simulink model "simulation"  (R2023b)
settings: Solver=FixedStepAuto  StartTime=0.0  StopTime=1e-6  FixedStep=1e-9  RelTol=1e-3
undefined symbols (not defined in the file): sigbuilder_block
libraries: fl_lib x47, nesl_utility x9, ee_lib x8
settings Model: Creator=Ryan  LastModifiedBy=shenjiarun
settings SolverCC: AlgebraicLoopSolver=TrustRegion
settings DebuggingCC: UnconnectedInputMsg=warning  UnconnectedOutputMsg=warning  UnconnectedLineMsg=warning
settings ModelReferenceCC: EnableRefExpFcnMdlSchedulingChecks=on
settings SFSimCC: CustomCodeUndefinedFunction=UseInterfaceOnly

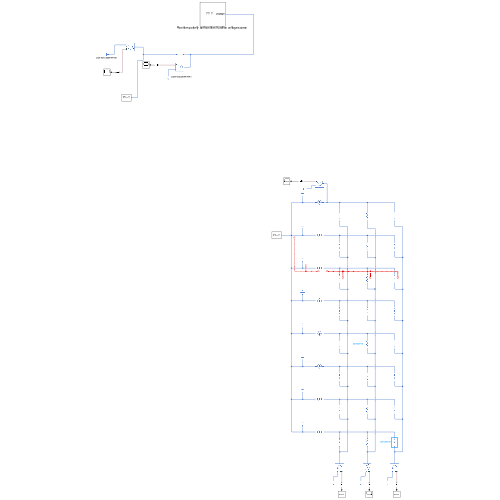
[thumbnail: Simulink's stored preview of the top-level diagram]
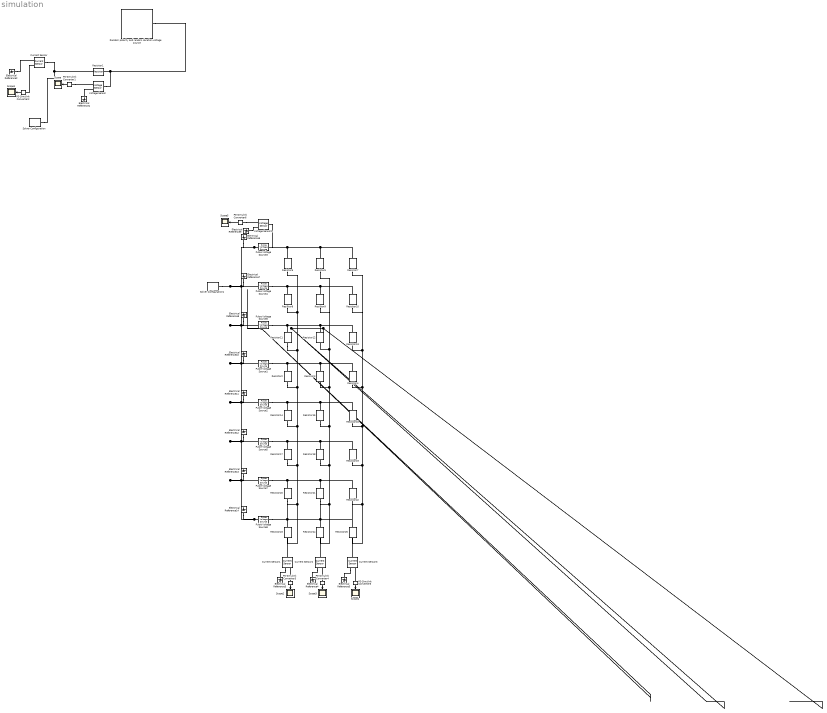
== system simulation ==
  Current Sensor{,1..3} (4 alike) : fl_lib/Electrical/Electrical Sensors/Current Sensor
  Electrical Reference{1..14} (14 alike) : fl_lib/Electrical/Electrical Elements/Electrical Reference
  PS-Simulink Converter{1..6} (6 alike) : nesl_utility/PS-Simulink Converter  PhysicalDomain=network_engine_domain  SubClassName=ps_output  LeftPortType=input  RightPortType=output  PseudoPeriodic=off  Frequencies=[]  VectorFormat=1-D array  Unit=1  AffineConversion=off
  Pulse Voltage Source{1,3,6,8} (4 alike) : ee_lib/Additional Components/SPICE Sources/Pulse Voltage Source  V1=0 V  V2=0.008 V  TD=0 s  TR=1e-9 s  TF=1e-9 s  PW=500e-9 s  PER=inf s
      settings: InternalSimscapePortConfiguration="{\"Bottom\":[],\"Left\":[{\"id\":\"p\",\"label\":\"\",\"type\":\"foundation.electrical.electrical\"}],\"Right\":[{\"id\":\"n\",\"label\":\"\",\"type\":\"foundation.electrical.electrical\"}],\"Top\":[]}"
  Pulse Voltage Source{2,4..5,7} (4 alike) : ee_lib/Additional Components/SPICE Sources/Pulse Voltage Source  V1=0 V  V2=0.2 V  TD=0 s  TR=1e-9 s  TF=1e-9 s  PW=500e-9 s  PER=inf s
      settings: InternalSimscapePortConfiguration="{\"Bottom\":[],\"Left\":[{\"id\":\"p\",\"label\":\"\",\"type\":\"foundation.electrical.electrical\"}],\"Right\":[{\"id\":\"n\",\"label\":\"\",\"type\":\"foundation.electrical.electrical\"}],\"Top\":[]}"
  Random polarity and random duration voltage source : Subsystem
      mask Display: image('D:\BaiduSyncdisk\UESTC\2022忆阻器萤火虫算法\论文写作\crossbar\随机.png');
  Resistor{1..3,5,7,9..11,13,16,18..19,22..25} (16 alike) : fl_lib/Electrical/Electrical Elements/Resistor  R=100 Ohm  i_specify=off  i_priority=None  i=0 A  i_nominal_specify=off  i_nominal_unit=A  i_nominal_value=1  v_specify=off  v_priority=None  v=0 V  v_nominal_specify=off  v_nominal_unit=V  v_nominal_value=1
  Resistor{4,6,8,12,14..15,17,20..21} (9 alike) : fl_lib/Electrical/Electrical Elements/Resistor  R=2500 Ohm  i_specify=off  i_priority=None  i=0 A  i_nominal_specify=off  i_nominal_unit=A  i_nominal_value=1  v_specify=off  v_priority=None  v=0 V  v_nominal_specify=off  v_nominal_unit=V  v_nominal_value=1
  Scope{,1..5} (6 alike) : Scope
  Solver Configuration : nesl_utility/Solver Configuration  PhysicalDomain=network_engine_domain  SubClassName=solver  LeftPortType=input  RightPortType=generic  Tones=[]  Harmonics=[]  SimulateNoise=off  Profile=off  UseLocalSampling=off  EnableSwitchedLinearOptims=on  FrequencyDomain=off  UseCCode=off  RelTol=0.001  AbsTol=1e-06  MinStep=1e-09  ToWorkspace=off  RevertToSquareIcSolve=off  NumHomotopyIterations=100  PhasorMode=off  PhasorModeNumHarmonics=1  ConsistencySolver=NEWTON_FTOL  IndexReductionMethod=DerivativeReplacement  DoDC=off  ResidualTolerance=1e-09  ConsistencyTolSource=GLOBAL  ConsistencyAbsTol=0.001  ConsistencyRelTol=0.001  ConsistencyTolFactor=0.001  UseLocalSolver=off  LocalSolverChoice=NE_BACKWARD_EULER_ADVANCER  ResolveIndetEquations=on  FunctionEvalNumThread=1  LocalSolverSampleTime=0.001  DoFixedCost=off  MaxNonlinIter=3  MaxModeIter=2  ComputeImpulses=off  ImpulseIterations=2  LinearAlgebra=auto  LinearAlgebraNumThread=0  EquationFormulation=NE_TIME_EF  DelaysMemoryBudget=1024  AutomaticFiltering=on  FilteringTimeConstant=0.001  PartitionStorageMethod=AS_NEEDED  PartitionMemoryBudget=1024  PartitionMethod=ROBUST  MultibodyUseLocalSolver=off  MultibodyLocalSolverChoice=ODE1  MultibodyLocalSolverSampleTime=0.001
  Solver Configuration1 : nesl_utility/Solver Configuration  PhysicalDomain=network_engine_domain  SubClassName=solver  LeftPortType=input  RightPortType=generic  Tones=[]  Harmonics=[]  SimulateNoise=off  Profile=off  UseLocalSampling=off  EnableSwitchedLinearOptims=on  FrequencyDomain=off  UseCCode=off  RelTol=0.001  AbsTol=1e-06  MinStep=1e-09  ToWorkspace=off  RevertToSquareIcSolve=off  NumHomotopyIterations=100  PhasorMode=off  PhasorModeNumHarmonics=1  ConsistencySolver=NEWTON_FTOL  IndexReductionMethod=DerivativeReplacement  DoDC=off  ResidualTolerance=1e-09  ConsistencyTolSource=GLOBAL  ConsistencyAbsTol=0.001  ConsistencyRelTol=0.001  ConsistencyTolFactor=0.001  UseLocalSolver=off  LocalSolverChoice=NE_BACKWARD_EULER_ADVANCER  ResolveIndetEquations=on  FunctionEvalNumThread=1  LocalSolverSampleTime=0.001  DoFixedCost=off  MaxNonlinIter=3  MaxModeIter=2  ComputeImpulses=off  ImpulseIterations=2  LinearAlgebra=auto  LinearAlgebraNumThread=0  EquationFormulation=NE_TIME_EF  DelaysMemoryBudget=1024  AutomaticFiltering=on  FilteringTimeConstant=0.001  PartitionStorageMethod=AS_NEEDED  PartitionMemoryBudget=1024  PartitionMethod=ROBUST  MultibodyUseLocalSolver=off  MultibodyLocalSolverChoice=ODE1  MultibodyLocalSolverSampleTime=0.001
  Voltage Sensor : fl_lib/Electrical/Electrical Sensors/Voltage Sensor
  Voltage Sensor1 : fl_lib/Electrical/Electrical Sensors/Voltage Sensor
  wires:
  PS-Simulink Converter1/1 -> Scope/1
  PS-Simulink Converter2/1 -> Scope1/1
  PS-Simulink Converter5/1 -> Scope4/1
  PS-Simulink Converter3/1 -> Scope2/1
  PS-Simulink Converter4/1 -> Scope3/1
  PS-Simulink Converter6/1 -> Scope5/1
  connections:
  Random polarity and random duration voltage source/RConn1 -- Voltage Sensor/LConn1 -- Resistor1/LConn1
  Solver Configuration/RConn1 -- Current Sensor/LConn1 -- Resistor1/RConn1
  Electrical Reference1/LConn1 -- Voltage Sensor/RConn2
  PS-Simulink Converter1/LConn1 -- Voltage Sensor/RConn1
  Electrical Reference2/LConn1 -- Current Sensor/RConn2
  PS-Simulink Converter2/LConn1 -- Current Sensor/RConn1
  Pulse Voltage Source8/RConn1 -- Solver Configuration1/RConn1 -- Electrical Reference7/LConn1 -- Pulse Voltage Source4/RConn1 -- Pulse Voltage Source3/RConn1 -- Electrical Reference6/LConn1 -- Electrical Reference8/LConn1 -- Pulse Voltage Source6/RConn1 -- Electrical Reference10/LConn1 -- Pulse Voltage Source1/RConn1 -- Electrical Reference11/LConn1 -- Pulse Voltage Source2/RConn1 -- Electrical Reference12/LConn1 -- Pulse Voltage Source5/RConn1 -- Electrical Reference13/LConn1 -- Pulse Voltage Source7/RConn1 -- Electrical Reference14/LConn1
  Resistor13/LConn1 -- Pulse Voltage Source6/LConn1 -- Resistor11/LConn1 -- Resistor12/LConn1
  Resistor6/LConn1 -- Resistor7/LConn1 -- Voltage Sensor1/LConn1 -- Pulse Voltage Source3/LConn1 -- Resistor5/LConn1
  Resistor9/LConn1 -- Resistor10/LConn1 -- Pulse Voltage Source4/LConn1 -- Resistor8/LConn1
  Resistor10/RConn1 -- Resistor7/RConn1 -- Current Sensor3/LConn1 -- Resistor25/RConn1 -- Resistor22/RConn1 -- Resistor19/RConn1 -- Resistor16/RConn1 -- Resistor4/RConn1 -- Resistor13/RConn1
  Resistor5/RConn1 -- Current Sensor1/LConn1 -- Resistor23/RConn1 -- Resistor20/RConn1 -- Resistor17/RConn1 -- Resistor14/RConn1 -- Resistor2/RConn1 -- Resistor11/RConn1 -- Resistor8/RConn1
  Resistor9/RConn1 -- Resistor6/RConn1 -- Current Sensor2/LConn1 -- Resistor24/RConn1 -- Resistor21/RConn1 -- Resistor18/RConn1 -- Resistor15/RConn1 -- Resistor3/RConn1 -- Resistor12/RConn1
  PS-Simulink Converter5/LConn1 -- Current Sensor3/RConn1
  PS-Simulink Converter3/LConn1 -- Current Sensor1/RConn1
  Current Sensor3/RConn2 -- Electrical Reference5/LConn1
  Current Sensor2/RConn2 -- Electrical Reference4/LConn1
  Current Sensor1/RConn2 -- Electrical Reference3/LConn1
  PS-Simulink Converter4/LConn1 -- Current Sensor2/RConn1
  Electrical Reference9/LConn1 -- Voltage Sensor1/RConn2
  PS-Simulink Converter6/LConn1 -- Voltage Sensor1/RConn1
  Resistor3/LConn1 -- Resistor4/LConn1 -- Pulse Voltage Source1/LConn1 -- Resistor2/LConn1
  Resistor15/LConn1 -- Resistor16/LConn1 -- Pulse Voltage Source2/LConn1 -- Resistor14/LConn1
  Resistor18/LConn1 -- Resistor19/LConn1 -- Pulse Voltage Source5/LConn1 -- Resistor17/LConn1
  Resistor21/LConn1 -- Resistor22/LConn1 -- Pulse Voltage Source7/LConn1 -- Resistor20/LConn1
  Resistor24/LConn1 -- Resistor25/LConn1 -- Pulse Voltage Source8/LConn1 -- Resistor23/LConn1
  ?
  ?
  ?
  ?
  ?
  ?

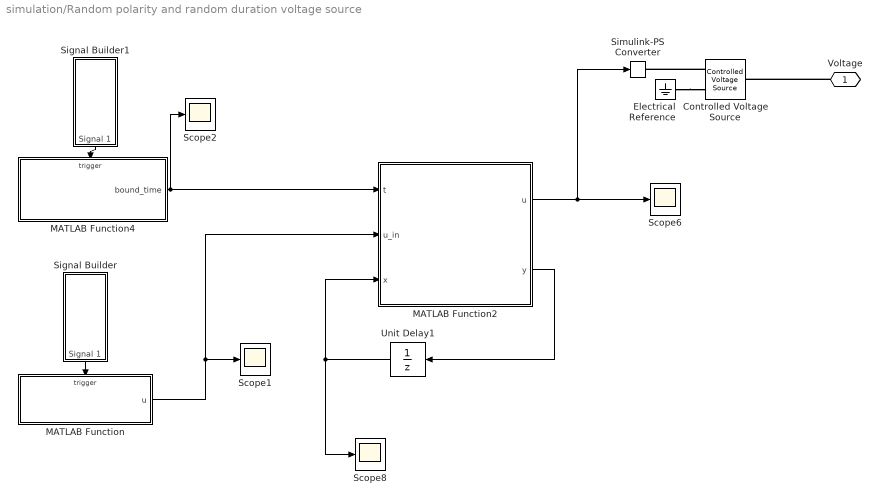
== system simulation/Random polarity and random duration voltage source ==
  Controlled Voltage Source : fl_lib/Electrical/Electrical Sources/Controlled Voltage Source
  Electrical Reference : fl_lib/Electrical/Electrical Elements/Electrical Reference
  MATLAB Function : MATLAB Function  TreatAsAtomicUnit=on
  MATLAB Function2 : MATLAB Function  TreatAsAtomicUnit=on
  MATLAB Function4 : MATLAB Function  TreatAsAtomicUnit=on
  Scope{1..2,6,8} (4 alike) : Scope
  Signal Builder : Subsystem  Tag=STV Subsys  LoadFcn=sigbuilder_block('load');  StartFcn=sigbuilder_block('start');  StopFcn=sigbuilder_block('stop');  ClipboardFcn=sigbuilder_block('clipboard');  mask(Sigbuilder block){tuvar=[0:10]}
      mask help: Simulink:masks:SigbuilderBlock_MD
      mask init:
      | if ~strcmp(get_param(bdroot(gcbh),'SimulationStatus'),'stopped') tuvar = sigbuilder_block('maskInit'); end
      settings: CopyFcn=sigbuilder_block('copy');  DeleteFcn=sigbuilder_block('delete');  ModelCloseFcn=sigbuilder_block('modelClose');  PreSaveFcn=sigbuilder_block('preSave');  PauseFcn=sigbuilder_block('pause');  ContinueFcn=sigbuilder_block('continue');  NameChangeFcn=sigbuilder_block('namechange');  OpenFcn=sigbuilder_block('open',[437.6 199.2 550.4 400 ]);  CloseFcn=sigbuilder_block('close');
      mask Display: plot(0, 0, 100, 100,[2, 2, 32, 32, 2], [68, 8, 8, 68, 68],[32, 2], [38, 38], [32, 19, 2],[53, 60, 44], [32, 17, 17, 2],[16, 16, 31, 31]);txt = getActiveGroup(gcbh);text(2, 100, txt,'verticalAlignment', 'top');
  Signal Builder1 : Subsystem  Tag=STV Subsys  LoadFcn=sigbuilder_block('load');  StartFcn=sigbuilder_block('start');  StopFcn=sigbuilder_block('stop');  ClipboardFcn=sigbuilder_block('clipboard');  mask(Sigbuilder block){tuvar=[0:10]}
      mask help: Simulink:masks:SigbuilderBlock_MD
      mask init:
      | if ~strcmp(get_param(bdroot(gcbh),'SimulationStatus'),'stopped') tuvar = sigbuilder_block('maskInit'); end
      settings: CopyFcn=sigbuilder_block('copy');  DeleteFcn=sigbuilder_block('delete');  ModelCloseFcn=sigbuilder_block('modelClose');  PreSaveFcn=sigbuilder_block('preSave');  PauseFcn=sigbuilder_block('pause');  ContinueFcn=sigbuilder_block('continue');  NameChangeFcn=sigbuilder_block('namechange');  OpenFcn=sigbuilder_block('open',[437.6 199.2 550.4 400 ]);  CloseFcn=sigbuilder_block('close');
      mask Display: plot(0, 0, 100, 100,[2, 2, 32, 32, 2], [68, 8, 8, 68, 68],[32, 2], [38, 38], [32, 19, 2],[53, 60, 44], [32, 17, 17, 2],[16, 16, 31, 31]);txt = getActiveGroup(gcbh);text(2, 100, txt,'verticalAlignment', 'top');
  Simulink-PS Converter : nesl_utility/Simulink-PS Converter  PhysicalDomain=network_engine_domain  SubClassName=ps_input  LeftPortType=input  RightPortType=output  PseudoPeriodic=off  Frequencies=[]  NoiseDistribution=none  NoiseParameters=[]  Unit=1  AffineConversion=off  FilteringAndDerivatives=provide  SimscapeFilterOrder=1  InputFilterTimeConstant=0.001  UdotUserProvided=0
  Unit Delay1 : UnitDelay  SampleTime=-1  HasFrameUpgradeWarning=on
  Voltage : PMIOPort  Side=Right
  wires:
  MATLAB Function/1(u) -> MATLAB Function2/2(u_in), Scope1/1
  Signal Builder/1(Signal 1) -> MATLAB Function/Trigger
  MATLAB Function2/1(u) -> Simulink-PS Converter/1, Scope6/1
  MATLAB Function2/2(y) -> Unit Delay1/1
  Unit Delay1/1 -> Scope8/1, MATLAB Function2/3(x)
  Signal Builder1/1(Signal 1) -> MATLAB Function4/Trigger
  MATLAB Function4/1(bound_time) -> MATLAB Function2/1(t), Scope2/1
  connections:
  Controlled Voltage Source/RConn1 -- Simulink-PS Converter/RConn1
  Electrical Reference/LConn1 -- Controlled Voltage Source/RConn2
  Voltage/RConn1 -- Controlled Voltage Source/LConn1

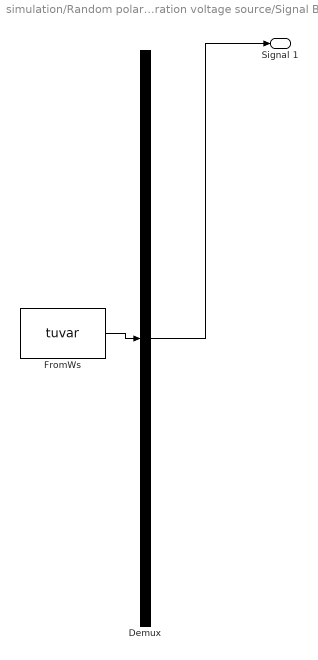
== system simulation/Random polarity and random duration voltage source/Signal Builder ==
  Demux : Demux  Tag=STV Demux  Outputs=1
      settings: DisplayOption=none
  FromWs : FromWorkspace  Tag=STV FromWs  VariableName=tuvar
      SigBuilderData=|
      | common.afterFinalStr = 'Extrapolate'
      | common.sampleTime = 0
      | dataSet.timeRange = [0 3e-09]
      | dataSet.name = 'Group 1'
      | sbobj.Groups.Name = 'Group 1'
      | sbobj.Groups.Signals.Name = 'Signal 1'
      | sbobj.Groups.Signals.XData = [0 2e-09 3e-09]
      | sbobj.Groups.Signals.YData = [0 -1 -1]
      | sbobj.Groups.TimeRange = [0 3e-09]
  Signal 1 : Outport  Tag=STV Outport  VectorParamsAs1DForOutWhenUnconnected=off
  wires:
  Demux/1 -> Signal 1/1
  FromWs/1 -> Demux/1

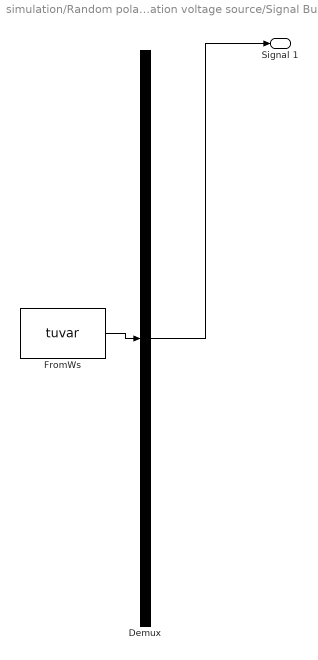
== system simulation/Random polarity and random duration voltage source/Signal Builder1 ==
  Demux : Demux  Tag=STV Demux  Outputs=1
      settings: DisplayOption=none
  FromWs : FromWorkspace  Tag=STV FromWs  VariableName=tuvar
      SigBuilderData=|
      | common.afterFinalStr = 'Extrapolate'
      | common.sampleTime = 0
      | dataSet.timeRange = [0 3e-09]
      | dataSet.name = 'Group 1'
      | sbobj.Groups.Name = 'Group 1'
      | sbobj.Groups.Signals.Name = 'Signal 1'
      | sbobj.Groups.Signals.XData = [0 2e-09 3e-09]
      | sbobj.Groups.Signals.YData = [0 -1 -1]
      | sbobj.Groups.TimeRange = [0 3e-09]
  Signal 1 : Outport  Tag=STV Outport  VectorParamsAs1DForOutWhenUnconnected=off
  wires:
  Demux/1 -> Signal 1/1
  FromWs/1 -> Demux/1

== matlab function simulation/Random polarity and random duration voltage source/MATLAB Function ==
  settings: sampleTime=1e-9
  data: u output
  events: trigger input EITHER_EDGE_EVENT
function u  = random_polarity
rand('seed', 10); %10----0.1291  1----0.5129
t = rand;
if t>=0.5
    u = 0.15;
else
    u = -0.15;
end
end

== matlab function simulation/Random polarity and random duration voltage source/MATLAB Function2 ==
  settings: sampleTime=1e-9
  data: t input; u_in input; u output; y output; x input
function [u,y] = timer(t, u_in, x)
x = x+1;
y = x;
if x>=t
    u=0
else
    u=u_in
end
end

== matlab function simulation/Random polarity and random duration voltage source/MATLAB Function4 ==
  settings: sampleTime=1e-9
  data: bound_time output
  events: trigger input EITHER_EDGE_EVENT
function bound_time  = time
rng('default');
rng(10);%设置种子
bound_time = randi([0,1000]);
end
